simulink model "Assignment_TestGen20"  (R2017b)
settings: Solver=FixedStepDiscrete  StartTime=0.0  StopTime=10.0  RelTol=1e-3
settings Model: Creator=hbourbou  LastModifiedBy=hbourbou
settings DebuggingCC: ParameterOverflowMsg=none

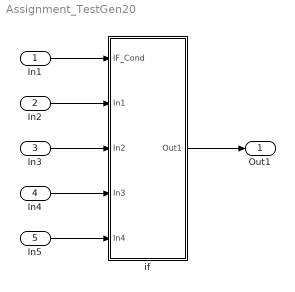
== system Assignment_TestGen20 ==
  In1 : Inport
  In2 : Inport  Port=2
  In3 : Inport  Port=3
  In4 : Inport  Port=4
  In5 : Inport  Port=5
  if : Subsystem  AncestorBlock=Block_TestLib/if
  Out1 : Outport
  wires:
  In1/1 -> if/1(IF_Cond)
  In2/1 -> if/2(In1)
  In3/1 -> if/3(In2)
  In4/1 -> if/4(In3)
  In5/1 -> if/5(In4)
  if/1(Out1) -> Out1/1

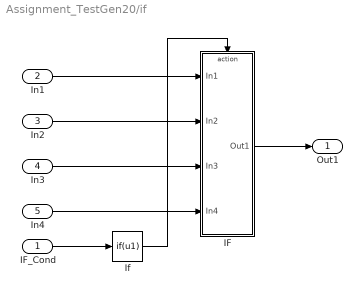
== system Assignment_TestGen20/if ==
  IF_Cond : Inport  OutDataTypeStr=boolean
  In1 : Inport  Port=2
  In2 : Inport  Port=3
  In3 : Inport  Port=4
  In4 : Inport  Port=5
  IF : Subsystem  TreatAsAtomicUnit=on
  If : If  IfExpression=u1  ShowElse=off
  Out1 : Outport
  wires:
  If/1 -> IF/Action
  In1/1 -> IF/1(In1)
  In2/1 -> IF/2(In2)
  In3/1 -> IF/3(In3)
  In4/1 -> IF/4(In4)
  IF_Cond/1 -> If/1
  IF/1(Out1) -> Out1/1

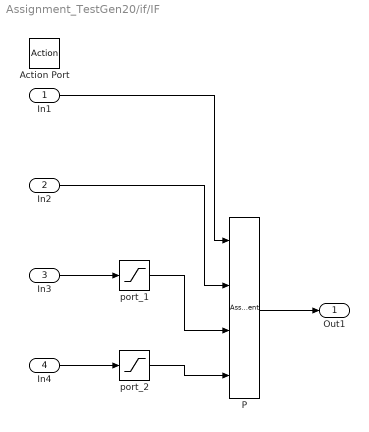
== system Assignment_TestGen20/if/IF ==
  In1 : Inport  OutDataTypeStr=int8  PortDimensions=[3 3 3 3]
  In2 : Inport  Port=2  OutDataTypeStr=int8  PortDimensions=[2 3 2 2]
  In3 : Inport  Port=3  OutMin=0  OutMax=1
  In4 : Inport  Port=4  OutMin=0  OutMax=1
  Action Port : ActionPort  ActionType=then
  P : Assignment  NumberOfDimensions=4  IndexMode=Zero-based  DiagnosticForDimensions=Warning  IndexOptions=Starting index (port),Assign all,Index vector (dialog),Index vector (port)  Indices=[],[],[1,2],[]  OutputSizes=,,,
  port_1 : Saturate  UpperLimit=1  LowerLimit=0
  port_2 : Saturate  UpperLimit=1  LowerLimit=0
  Out1 : Outport
  wires:
  In1/1 -> P/1
  In2/1 -> P/2
  port_1/1 -> P/3
  port_2/1 -> P/4
  In3/1 -> port_1/1
  In4/1 -> port_2/1
  P/1 -> Out1/1
